simulink model "FOC08022311"  (R2025a)
settings: Solver=FixedStepAuto  StartTime=0.0  StopTime=1  RelTol=1e-3
values from neighbouring files (symbols this model uses):
  B = 0    [FOC08022311parameters.m]
  f_n = 50    [FOC08022311parameters.m]
  flux_n = L_m * Ids_n    [FOC08022311parameters.m]
  Ids_n = V_max / sqrt(R_s^2 + (w_n * L_s)^2)    [FOC08022311parameters.m]
  J = 0.1284    [FOC08022311parameters.m]
  ka_i = 1 / kp_i    (= 0.0140032473775)    [FOC08022311parameters.m]
  ki_i = R * wc_i    (= 19541.6337915)    [FOC08022311parameters.m]
  kp_i = L * wc_i    (= 71.4120070181)    [FOC08022311parameters.m]
  L_lr = 0.2898-0.2838    (= 0.006)    [FOC08022311parameters.m]
  L_ls = 0.294-0.2838    (= 0.0102)    [FOC08022311parameters.m]
  L_m = 1*0.2838    (= 0.2838)    [FOC08022311parameters.m]
  L_r = L_m + L_lr    (= 0.2898)    [FOC08022311parameters.m]
  L_s = L_m + L_ls    (= 0.294)    [FOC08022311parameters.m]
  n_p = 2    [FOC08022311parameters.m]
  P_n = 3000    [FOC08022311parameters.m]
  R_r = 2.658    [FOC08022311parameters.m]
  R_s = 1.85    [FOC08022311parameters.m]
  rpm_n = 1400    [FOC08022311parameters.m]
  sigma = 1 - L_m^2 / (L_s * L_r)    (= 0.0546795115562)    [FOC08022311parameters.m]
  T_r = L_r / R_r    (= 0.109029345372)    [FOC08022311parameters.m]
  T_sw = 1 / f_sw    (= 0.0001)    [FOC08022311parameters.m]
  V_dc = 500    [FOC08022311parameters.m]
  V_max = V_n * sqrt(2) / sqrt(3)    [FOC08022311parameters.m]
  V_n = 380    [FOC08022311parameters.m]
libraries: simulink x3, slpidlib x2, spsAsynchronousMachineSIUnitsLib x1, spsDCVoltageSourceLib x1, spsAlphaBetaZerotoabcLib x1, spsTriangleGeneratorLib x1, spsUniversalBridgeLib x1, spsabctodq0Lib x1, spsdq0toAlphaBetaZeroLib x1, spspowerguiLib x1
settings Model: Creator=11048  LastModifiedBy=ASUS
settings RTWCC: GPUComputeCapability=3.5

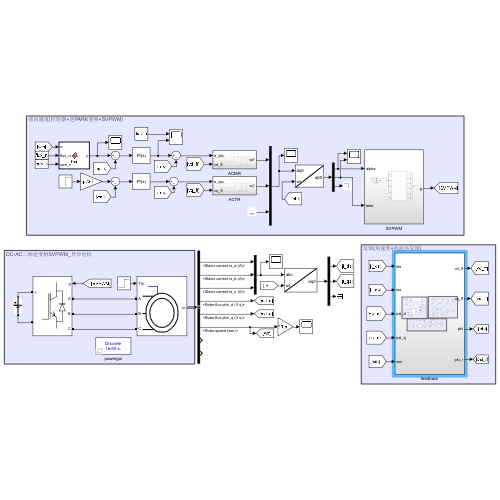
[thumbnail: Simulink's stored preview of the top-level diagram]
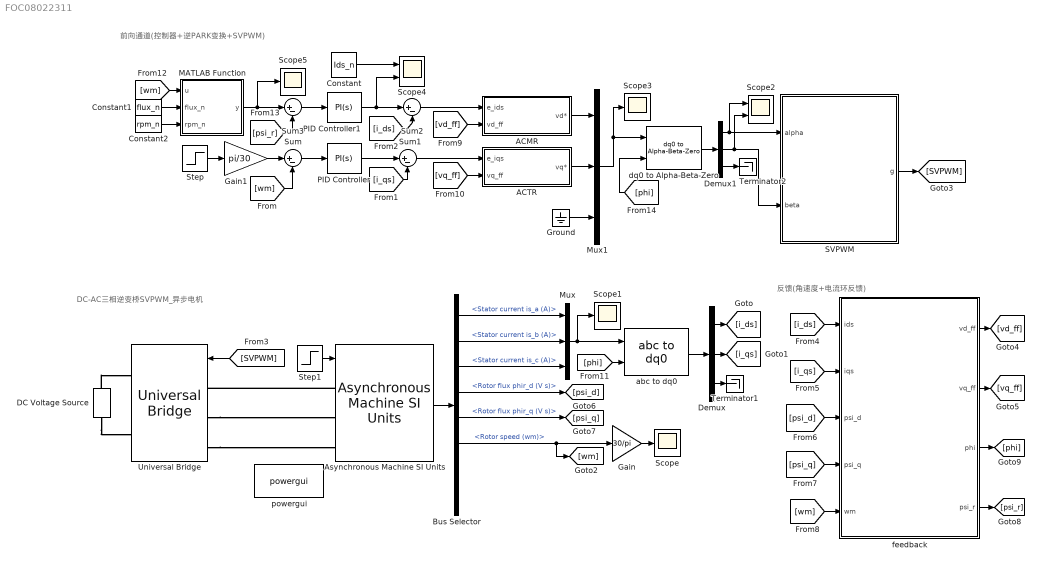
== system FOC08022311 ==
  note: 反馈(角速度+电流环反馈)
  note: 前向通道(控制器+逆PARK变换+SVPWM)
  note: DC-AC三相逆变桥SVPWM_异步电机
  ACMR : Subsystem
  ACTR : Subsystem
  Asynchronous Machine SI Units : spsAsynchronousMachineSIUnitsLib/Asynchronous Machine SI Units  RotorType=Squirrel-cage  PresetModel=No  MechanicalLoad=Torque Tm  ShowDetailedParameters=on  ReferenceFrame=Stationary  Units=SI  MeasurementBus=off  NominalParameters=[P_n V_n f_n]  VoltageRatio=1  Stator=[R_s L_ls]  Rotor=[R_r L_lr]  Cage1=[0.4155 0.002066]  Cage2=[0.4168 0.0003495]  Lm=L_m  Mechanical=[J B n_p]  PolePairs=2  InitialConditions=[1 0 0 0 0 0 0 0]  SimulateSaturation=off  Saturation=[14.03593122, 27.81365428, 53.79336849, 72.68890987, 97.98006896, 148.6815601, 215.7428561, 302.9841135, 428.7778367 ; 230, 322, 414, 460, 506, 552, 598, 644, 690]  LoadFlowParameters=1492000  TsPowergui=0  TsBlock=-1  IterativeModel=Trapezoidal non iterative  IterativeDiscreteModel=Trapezoidal non iterative  Pmec=1.492e+006
  Bus Selector : BusSelector  OutputSignals=Stator measurements.Stator current is_a (A),Stator measurements.Stator current is_b (A),Stator measurements.Stator current is_c (A),Rotor measurements.Rotor flux phir_d (V s),Rotor measurements.Rotor flux phir_q (V s),Mechanical.Rotor speed (wm),Mechanical.Electromagnetic torque Te (N*m),Mechanical.Rotor angle thetam (rad)
  Constant : Constant  Value=Ids_n
  Constant1 : Constant  Value=flux_n
  Constant2 : Constant  Value=rpm_n
  DC Voltage Source : spsDCVoltageSourceLib/DC Voltage Source  Amplitude=V_dc  Measurements=None
  Demux : Demux  Outputs=3
  Demux1 : Demux  Outputs=3
  Gain : Gain  Gain=30/pi
  Gain1 : Gain  Gain=pi/30
  Ground : Ground
  MATLAB Function : MATLAB Function  TreatAsAtomicUnit=on
  Mux : Mux  Inputs=3
  Mux1 : Mux  Inputs=3
  PID Controller : slpidlib/PID Controller  Controller=PI  Form=Parallel  TimeDomain=Continuous-time  UseExternalTs=off  SampleTime=-1  IntegratorMethod=Forward Euler  FilterMethod=Forward Euler  ControllerParametersSource=internal  P=20  I=1.5  UseKiTs=off  D=0  UseExternalDerivativeSource=off  N=100  UseFilter=on  TunerSelectOption=Transfer Function Based (PID Tuner App)  InitialConditionSource=internal  InitialConditionForIntegrator=0  InitialConditionForFilter=0  DifferentiatorICPrevScaledInput=0  ExternalReset=none  TrackingMode=off  Kt=1  LimitOutput=off  SatLimitsSource=internal  UpperSaturationLimit=inf  LowerSaturationLimit=-inf  LinearizeAsGain=on  AntiWindupMode=none  Kb=1  LimitIntegrator=off  UpperIntegratorSaturationLimit=inf  LowerIntegratorSaturationLimit=-inf  POutMin=[]  POutMax=[]  IOutMin=[]  IOutMax=[]  DOutMin=[]  DOutMax=[]  NOutMin=[]  NOutMax=[]  SumOutMin=[]  SumOutMax=[]  SaturationOutMin=[]  SaturationOutMax=[]  PParamMin=[]  PParamMax=[]  IParamMin=[]  IParamMax=[]  DParamMin=[]  DParamMax=[]  NParamMin=[]  NParamMax=[]  KbParamMin=[]  KbParamMax=[]  KtParamMin=[]  KtParamMax=[]  KbOutMin=[]  KbOutMax=[]  KtOutMin=[]  KtOutMax=[]  IntegratorOutMin=[]  IntegratorOutMax=[]  FilterOutMin=[]  FilterOutMax=[]  SumI1OutMin=[]  SumI1OutMax=[]  SumI2OutMin=[]  SumI2OutMax=[]  SumI3OutMin=[]  SumI3OutMax=[]  SumI4OutMin=[]  SumI4OutMax=[]  SumDOutMin=[]  SumDOutMax=[]  DifferentiatorOutMin=[]  DifferentiatorOutMax=[]  FilterDiffOutCoefMin=[]  FilterDiffOutCoefMax=[]  ReciprocalOutMin=[]  ReciprocalOutMax=[]  SumDenOutMin=[]  SumDenOutMax=[]  SumNumOutMin=[]  SumNumOutMax=[]  DivideOutMin=[]  DivideOutMax=[]  UdiffTsProdOutMin=[]  UdiffTsProdOutMax=[]  NTsProdOutMin=[]  NTsProdOutMax=[]  UintegralTsProdOutMin=[]  UintegralTsProdOutMax=[]  UngainTsProdOutMin=[]  UngainTsProdOutMax=[]  ClampingZeroOutDataTypeStr=Inherit: Inherit via back propagation  ClampingZeroOutMin=[]  ClampingZeroOutMax=[]  FilterDenConstantOutDataTypeStr=Inherit: Inherit via back propagation  FilterDenConstantOutMin=[]  FilterDenConstantOutMax=[]  PCopyOutDataTypeStr=Inherit: Inherit via back propagation  PCopyOutMin=[]  PCopyOutMax=[]  NCopyOutDataTypeStr=Inherit: Inherit via back propagation  NCopyOutMin=[]  NCopyOutMax=[]  IntegratorContinuousStateAttributes=''  IntegratorStateMustResolveToSignalObject=off  IntegratorRTWStateStorageClass=Auto  FilterContinuousStateAttributes=''  FilterStateMustResolveToSignalObject=off  FilterRTWStateStorageClass=Auto  ParallelPVariant=InternalParameters  IdealPVariant=Disabled  IVariant=InternalParameters  DVariant=Disabled  IntegratorVariant=Continuous  SatVariant=Disabled  AWVariant=Passthrough  PCopyVariant=Disabled  TRVariant=Disabled  FdbkBlocksVariant=Forward  IdealPFdbkVariant=Disabled  SatFdbkVariant=Disabled  DerivativeFilterVariant=Disabled  NVariant=Disabled  NCopyVariant=Disabled_SignalSpec  FilterICVariant=Disabled  IntegratorICVariant=InternalICs  ExternalResetVariant=Disabled  TRSumVariant=Passthrough  SumFdbkVariant=Disabled  SumVariant=Sum_PI  TsampFilterVariant=InternalTs  TsampNgainVariant=Passthrough  TsampIntegralVariant=Disabled_SignalSpec  ExternalSaturationOutDataTypeStr=Inherit: Same as second input  DerivativeSourceVariant=Disabled  PreIntVariant=InternalPreInt
  PID Controller1 : slpidlib/PID Controller  Controller=PI  Form=Parallel  TimeDomain=Continuous-time  UseExternalTs=off  SampleTime=-1  IntegratorMethod=Forward Euler  FilterMethod=Forward Euler  ControllerParametersSource=internal  P=1/L_m  I=5  UseKiTs=off  D=0  UseExternalDerivativeSource=off  N=100  UseFilter=on  TunerSelectOption=Transfer Function Based (PID Tuner App)  InitialConditionSource=internal  InitialConditionForIntegrator=0  InitialConditionForFilter=0  DifferentiatorICPrevScaledInput=0  ExternalReset=none  TrackingMode=off  Kt=1  LimitOutput=off  SatLimitsSource=internal  UpperSaturationLimit=inf  LowerSaturationLimit=-inf  LinearizeAsGain=on  AntiWindupMode=none  Kb=1  LimitIntegrator=off  UpperIntegratorSaturationLimit=inf  LowerIntegratorSaturationLimit=-inf  POutMin=[]  POutMax=[]  IOutMin=[]  IOutMax=[]  DOutMin=[]  DOutMax=[]  NOutMin=[]  NOutMax=[]  SumOutMin=[]  SumOutMax=[]  SaturationOutMin=[]  SaturationOutMax=[]  PParamMin=[]  PParamMax=[]  IParamMin=[]  IParamMax=[]  DParamMin=[]  DParamMax=[]  NParamMin=[]  NParamMax=[]  KbParamMin=[]  KbParamMax=[]  KtParamMin=[]  KtParamMax=[]  KbOutMin=[]  KbOutMax=[]  KtOutMin=[]  KtOutMax=[]  IntegratorOutMin=[]  IntegratorOutMax=[]  FilterOutMin=[]  FilterOutMax=[]  SumI1OutMin=[]  SumI1OutMax=[]  SumI2OutMin=[]  SumI2OutMax=[]  SumI3OutMin=[]  SumI3OutMax=[]  SumI4OutMin=[]  SumI4OutMax=[]  SumDOutMin=[]  SumDOutMax=[]  DifferentiatorOutMin=[]  DifferentiatorOutMax=[]  FilterDiffOutCoefMin=[]  FilterDiffOutCoefMax=[]  ReciprocalOutMin=[]  ReciprocalOutMax=[]  SumDenOutMin=[]  SumDenOutMax=[]  SumNumOutMin=[]  SumNumOutMax=[]  DivideOutMin=[]  DivideOutMax=[]  UdiffTsProdOutMin=[]  UdiffTsProdOutMax=[]  NTsProdOutMin=[]  NTsProdOutMax=[]  UintegralTsProdOutMin=[]  UintegralTsProdOutMax=[]  UngainTsProdOutMin=[]  UngainTsProdOutMax=[]  ClampingZeroOutDataTypeStr=Inherit: Inherit via back propagation  ClampingZeroOutMin=[]  ClampingZeroOutMax=[]  FilterDenConstantOutDataTypeStr=Inherit: Inherit via back propagation  FilterDenConstantOutMin=[]  FilterDenConstantOutMax=[]  PCopyOutDataTypeStr=Inherit: Inherit via back propagation  PCopyOutMin=[]  PCopyOutMax=[]  NCopyOutDataTypeStr=Inherit: Inherit via back propagation  NCopyOutMin=[]  NCopyOutMax=[]  IntegratorContinuousStateAttributes=''  IntegratorStateMustResolveToSignalObject=off  IntegratorRTWStateStorageClass=Auto  FilterContinuousStateAttributes=''  FilterStateMustResolveToSignalObject=off  FilterRTWStateStorageClass=Auto  ParallelPVariant=InternalParameters  IdealPVariant=Disabled  IVariant=InternalParameters  DVariant=Disabled  IntegratorVariant=Continuous  SatVariant=Disabled  AWVariant=Passthrough  PCopyVariant=Disabled  TRVariant=Disabled  FdbkBlocksVariant=Forward  IdealPFdbkVariant=Disabled  SatFdbkVariant=Disabled  DerivativeFilterVariant=Disabled  NVariant=Disabled  NCopyVariant=Disabled_SignalSpec  FilterICVariant=Disabled  IntegratorICVariant=InternalICs  ExternalResetVariant=Disabled  TRSumVariant=Passthrough  SumFdbkVariant=Disabled  SumVariant=Sum_PI  TsampFilterVariant=InternalTs  TsampNgainVariant=Passthrough  TsampIntegralVariant=Disabled_SignalSpec  ExternalSaturationOutDataTypeStr=Inherit: Same as second input  DerivativeSourceVariant=Disabled  PreIntVariant=InternalPreInt
  SVPWM : Subsystem
  Scope{,1,3,5} (4 alike) : Scope
      Scope settings: ActiveDisplayYMinimum=-245.05423330740308  ActiveDisplayYMaximum=2182.1289862079198
      Scope1 settings: ActiveDisplayYMinimum=-1  ActiveDisplayYMaximum=1  DataLoggingVariableName=ScopeData2
      Scope3 settings: ActiveDisplayYMinimum=-553.80143526649249  ActiveDisplayYMaximum=499.74368491943784
      Scope5 settings: ActiveDisplayYMinimum=0.877559064610581  ActiveDisplayYMaximum=0.96156070598738208  DataLoggingVariableName=ScopeData9
  Scope2 : Scope  NumInputPorts=2
      settings: ActiveDisplayYMinimum=-1  ActiveDisplayYMaximum=1  DataLoggingVariableName=ScopeData5
  Scope4 : Scope  NumInputPorts=2
      settings: ActiveDisplayYMinimum=-2.7427305612345254  ActiveDisplayYMaximum=4.03663172867287  DataLoggingVariableName=ScopeData8
  Step : Step  Time=0.6  Before=1000  After=1500  SampleTime=0
  Step1 : Step  Time=0.3  Before=10  After=20  SampleTime=0
  Sum{,1..3} (4 alike) : Sum  Inputs=|+-
  Terminator1 : Terminator
  Terminator2 : Terminator
  Universal Bridge : spsUniversalBridgeLib/Universal Bridge  Arms=3  SnubberResistance=1e5  SnubberCapacitance=inf  Device=IGBT / Diodes  Ron=1e-3  Lon=0  ForwardVoltages="[  0  0  ]"  ForwardVoltage=0  GTOparameters=[ 10e-6 , 20e-6 ]  IGBTparameters=[ 1e-6 , 2e-6 ]  Measurements=None  Measurements_2=None  converterType=Rectifier
  abc to dq0 : spsabctodq0Lib/abc to dq0  Alignment=90 degrees behind phase A axis
  dq0 to Alpha-Beta-Zero : spsdq0toAlphaBetaZeroLib/dq0 to Alpha-Beta-Zero  Alignment=90 degrees behind phase A axis
  feedback : Subsystem
  powergui : spspowerguiLib/powergui  Priority=1  SimulationMode=Discrete  SampleTime=T_sw/10  frequency=60  Iterations=50  frequencyindice=50  Pbase=100e6  ErrMax=1e-4  UnitsV=kV  UnitsW=MW  buscounter=0  FunctionMessages=off  echomessages=off  EnableUseOfTLC=off  CurrentSourceSwitches=off  DisableSnubberDevices=off  DisableRonSwitches=off  DisableVfSwitches=off  DisplayEquations=off  AutomaticDiscreteSolvers=off  SolverType=Tustin/Backward Euler (TBE)  Interpol=off  ExternalGateDelay=off  methode=off  Ts=100  x0status=blocks  SPID=on  SwTol=0  HookPort=off  NonlinearTolerance=1e-4  nMaxIteration=100  ContinueOnMaxIteration=off  RestoreLinks=warning  ResistiveCurrentMeasurement=off  Frange=[0:2:500]  Ylog=off  Xlog=on  ShowGrid=off  save=off  variable=ZData  structure=0  ZoomFFT=off  StartTime=0.0  cycles=1  DisplayStyle=1  fundamental=60  FreqAxis=off  MaxFrequency=1000  frequencyindicesteady=1  RmsSteady=1  display=off
  wires:
  Asynchronous Machine SI Units/1 -> Bus Selector/1
  Bus Selector/4 -> [psi_d]  "<Rotor flux phir_d (V s)>"
  Bus Selector/1 -> Mux/1  "<Stator current is_a (A)>"
  Bus Selector/2 -> Mux/2  "<Stator current is_b (A)>"
  Bus Selector/3 -> Mux/3  "<Stator current is_c (A)>"
  Bus Selector/6 -> Gain/1, [wm]  "<Rotor speed (wm)>"
  Gain/1 -> Scope/1
  Step/1 -> Gain1/1
  Gain1/1 -> Sum/1
  [wm] -> Sum/2
  Sum/1 -> PID Controller/1
  PID Controller/1 -> Sum1/1
  [i_qs] -> Sum1/2
  Sum1/1 -> ACTR/1(e_iqs)
  [i_ds] -> Sum2/2
  Sum2/1 -> ACMR/1(e_ids)
  Mux1/1 -> dq0 to Alpha-Beta-Zero/1, Scope3/1
  dq0 to Alpha-Beta-Zero/1 -> Demux1/1
  Demux1/3 -> Terminator2/1
  [SVPWM] -> Universal Bridge/1
  feedback/2(vq_ff) -> [vq_ff]
  [i_qs] -> feedback/2(iqs)
  [psi_d] -> feedback/3(psi_d)
  [psi_q] -> feedback/4(psi_q)
  [wm] -> feedback/5(wm)
  [vq_ff] -> ACTR/2(vq_ff)
  [vd_ff] -> ACMR/2(vd_ff)
  Step1/1 -> Asynchronous Machine SI Units/1
  SVPWM/1(g) -> [SVPWM]
  Demux/3 -> Terminator1/1
  Demux/1 -> [i_ds]
  Demux/2 -> [i_qs]
  abc to dq0/1 -> Demux/1
  [phi] -> abc to dq0/2
  Mux/1 -> abc to dq0/1, Scope1/1
  Bus Selector/5 -> [psi_q]  "<Rotor flux phir_q (V s)>"
  [i_ds] -> feedback/1(ids)
  [phi] -> dq0 to Alpha-Beta-Zero/2
  Demux1/1 -> SVPWM/1(alpha), Scope2/1
  Demux1/2 -> SVPWM/2(beta), Scope2/2
  feedback/3(phi) -> [phi]
  Ground/1 -> Mux1/3
  ACMR/1(vd*) -> Mux1/1
  ACTR/1(vq*) -> Mux1/2
  feedback/1(vd_ff) -> [vd_ff]
  PID Controller1/1 -> Scope4/2, Sum2/1
  [wm] -> MATLAB Function/1(u)
  feedback/4(psi_r) -> [psi_r]
  [psi_r] -> Sum3/2
  MATLAB Function/1(y) -> Scope5/1, Sum3/1
  Sum3/1 -> PID Controller1/1
  Constant1/1 -> MATLAB Function/2(flux_n)
  Constant2/1 -> MATLAB Function/3(rpm_n)
  Constant/1 -> Scope4/1
  connections:
  DC Voltage Source/RConn1 -- Universal Bridge/RConn1
  DC Voltage Source/LConn1 -- Universal Bridge/RConn2
  Asynchronous Machine SI Units/LConn1 -- Universal Bridge/LConn1
  Universal Bridge/LConn2 -- Asynchronous Machine SI Units/LConn2
  Universal Bridge/LConn3 -- Asynchronous Machine SI Units/LConn3

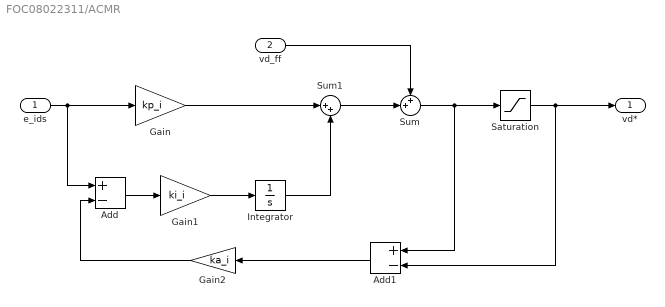
== system FOC08022311/ACMR ==
  e_ids : Inport
  vd_ff : Inport  Port=2
  Add : Sum  Inputs=+-
  Add1 : Sum  Inputs=+-
  Gain : Gain  Gain=kp_i
  Gain1 : Gain  Gain=ki_i
  Gain2 : Gain  Gain=ka_i
  Integrator : Integrator
  Saturation : Saturate  UpperLimit=V_max * 2  LowerLimit=-V_max * 2
  Sum : Sum  Inputs=++|
  Sum1 : Sum  Inputs=|++
  vd* : Outport
  wires:
  Gain2/1 -> Add/2
  Add1/1 -> Gain2/1
  Saturation/1 -> vd*/1, Add1/2
  Sum/1 -> Saturation/1, Add1/1
  Add/1 -> Gain1/1
  e_ids/1 -> Add/1, Gain/1
  vd_ff/1 -> Sum/1
  Integrator/1 -> Sum1/2
  Gain/1 -> Sum1/1
  Sum1/1 -> Sum/2
  Gain1/1 -> Integrator/1

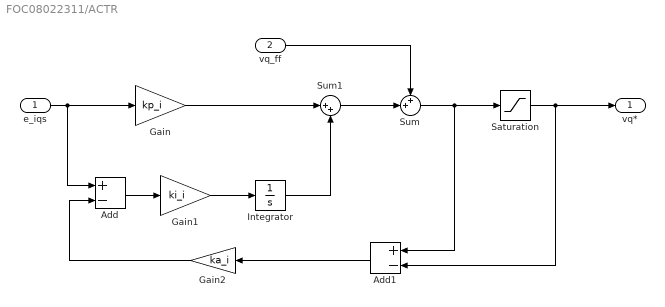
== system FOC08022311/ACTR ==
  e_iqs : Inport
  vq_ff : Inport  Port=2
  Add : Sum  Inputs=+-
  Add1 : Sum  Inputs=+-
  Gain : Gain  Gain=kp_i
  Gain1 : Gain  Gain=ki_i
  Gain2 : Gain  Gain=ka_i
  Integrator : Integrator
  Saturation : Saturate  UpperLimit=V_max*2  LowerLimit=-V_max * 2
  Sum : Sum  Inputs=++|
  Sum1 : Sum  Inputs=|++
  vq* : Outport
  wires:
  Gain1/1 -> Integrator/1
  Sum1/1 -> Sum/2
  Gain/1 -> Sum1/1
  Integrator/1 -> Sum1/2
  vq_ff/1 -> Sum/1
  e_iqs/1 -> Gain/1, Add/1
  Add/1 -> Gain1/1
  Sum/1 -> Add1/1, Saturation/1
  Saturation/1 -> Add1/2, vq*/1
  Add1/1 -> Gain2/1
  Gain2/1 -> Add/2

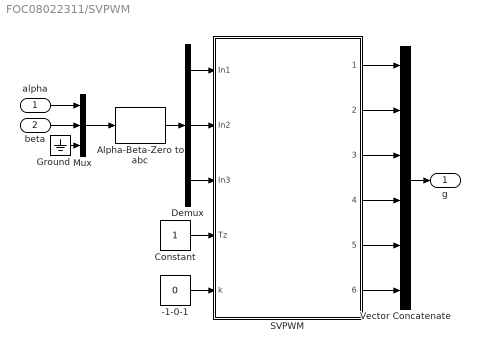
== system FOC08022311/SVPWM ==
  alpha : Inport
  beta : Inport  Port=2
  -1-0-1 : Constant  Value=0
  Alpha-Beta-Zero to abc : spsAlphaBetaZerotoabcLib/Alpha-Beta-Zero to abc
      settings: LibrarySourceBlock=|
      | sps_lib/Control/Alpha-Beta-Zero
      | to abc
  Constant : Constant
  Demux : Demux  Outputs=3
  Ground : Ground
  Mux : Mux  Inputs=3
  SVPWM : Subsystem
  Vector Concatenate : Concatenate  NumInputs=6
  g : Outport
  wires:
  alpha/1 -> Mux/1
  beta/1 -> Mux/2
  SVPWM/5(5) -> Vector Concatenate/5
  SVPWM/4(4) -> Vector Concatenate/4
  Demux/2 -> SVPWM/2(In2)
  -1-0-1/1 -> SVPWM/5(k)
  SVPWM/6(6) -> Vector Concatenate/6
  Constant/1 -> SVPWM/4(Tz)
  SVPWM/2(2) -> Vector Concatenate/2
  Demux/3 -> SVPWM/3(In3)
  SVPWM/1(1) -> Vector Concatenate/1
  Demux/1 -> SVPWM/1(In1)
  SVPWM/3(3) -> Vector Concatenate/3
  Vector Concatenate/1 -> g/1
  Mux/1 -> Alpha-Beta-Zero to abc/1
  Alpha-Beta-Zero to abc/1 -> Demux/1
  Ground/1 -> Mux/3

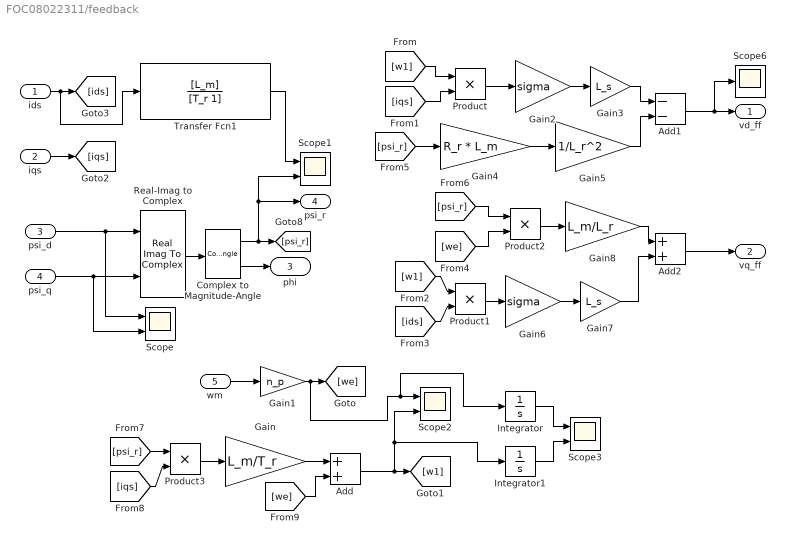
== system FOC08022311/feedback ==
  ids : Inport
  iqs : Inport  Port=2
  psi_d : Inport  Port=3
  psi_q : Inport  Port=4
  wm : Inport  Port=5
  Add : Sum
  Add1 : Sum  Inputs=--
  Add2 : Sum
  Complex to Magnitude-Angle : ComplexToMagnitudeAngle
  Gain : Gain  Gain=L_m/T_r
  Gain1 : Gain  Gain=n_p
  Gain2 : Gain  Gain=sigma
  Gain3 : Gain  Gain=L_s
  Gain4 : Gain  Gain=R_r * L_m
  Gain5 : Gain  Gain=1/L_r^2
  Gain6 : Gain  Gain=sigma
  Gain7 : Gain  Gain=L_s
  Gain8 : Gain  Gain=L_m/L_r
  Integrator : Integrator
  Integrator1 : Integrator
  Product{,1..3} (4 alike) : Product
  Real-Imag to Complex : RealImagToComplex
  Scope{,1..3} (4 alike) : Scope  NumInputPorts=2
      Scope settings: ActiveDisplayYMinimum=-1.6110842776276593  ActiveDisplayYMaximum=1.5992338688221852  DataLoggingVariableName=ScopeData7
      Scope1 settings: ActiveDisplayYMinimum=-0.19199842830712538  ActiveDisplayYMaximum=1.7279858547641289  DataLoggingVariableName=ScopeData3
      Scope2 settings: ActiveDisplayYMinimum=-28.950143898994849  ActiveDisplayYMaximum=260.34761589561333  DataLoggingVariableName=ScopeData4
      Scope3 settings: ActiveDisplayYMinimum=-1  ActiveDisplayYMaximum=1  DataLoggingVariableName=ScopeData6
  Scope6 : Scope
      settings: ActiveDisplayYMinimum=-1  ActiveDisplayYMaximum=1  DataLoggingVariableName=usm0601  DataLoggingSaveFormat=Array
  Transfer Fcn1 : TransferFcn  Numerator=[L_m]  Denominator=[T_r 1]
  vd_ff : Outport
  vq_ff : Outport  Port=2
  phi : Outport  Port=3
  psi_r : Outport  Port=4
  wires:
  ids/1 -> Transfer Fcn1/1, [ids]
  iqs/1 -> [iqs]
  Gain/1 -> Add/1
  wm/1 -> Gain1/1
  Gain1/1 -> Integrator/1, Scope2/1, [we]
  Add/1 -> Integrator1/1, Scope2/2, [w1]
  [w1] -> Product/1
  [iqs] -> Product/2
  Product/1 -> Gain2/1
  Gain2/1 -> Gain3/1
  Gain4/1 -> Gain5/1
  Gain3/1 -> Add1/1
  Gain5/1 -> Add1/2
  Add1/1 -> vd_ff/1, Scope6/1
  Gain6/1 -> Gain7/1
  [w1] -> Product1/1
  Product1/1 -> Gain6/1
  [ids] -> Product1/2
  [we] -> Product2/2
  Product2/1 -> Gain8/1
  Gain8/1 -> Add2/1
  Gain7/1 -> Add2/2
  Add2/1 -> vq_ff/1
  psi_d/1 -> Real-Imag to Complex/1, Scope/1
  Real-Imag to Complex/1 -> Complex to Magnitude-Angle/1
  Complex to Magnitude-Angle/2 -> phi/1
  Complex to Magnitude-Angle/1 -> psi_r/1, Scope1/2, [psi_r]
  psi_q/1 -> Scope/2, Real-Imag to Complex/2
  Product3/1 -> Gain/1
  [psi_r] -> Gain4/1
  [psi_r] -> Product2/1
  [psi_r] -> Product3/1
  [iqs] -> Product3/2
  [we] -> Add/2
  Transfer Fcn1/1 -> Scope1/1
  Integrator/1 -> Scope3/1
  Integrator1/1 -> Scope3/2

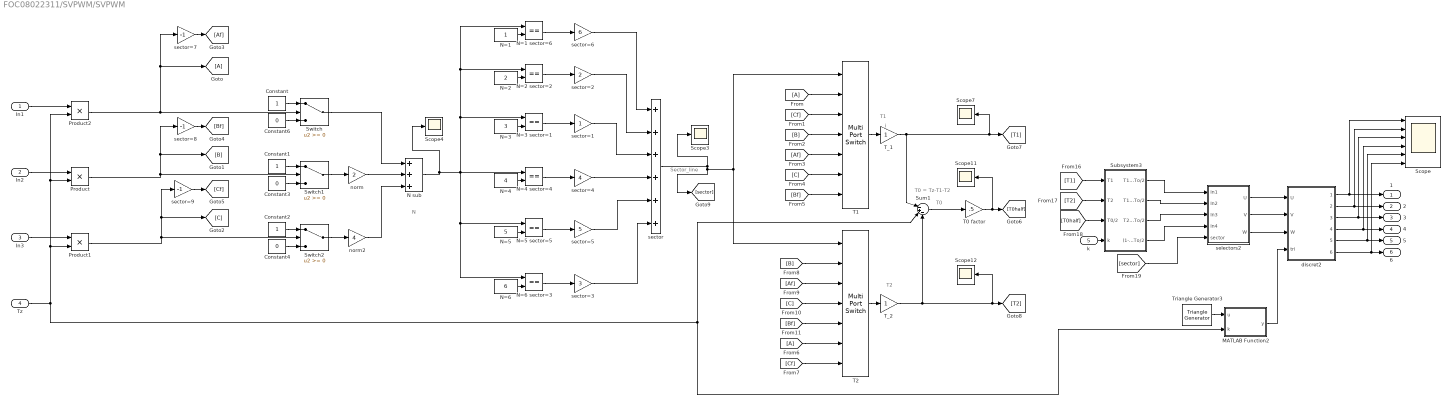
== system FOC08022311/SVPWM/SVPWM ==
  note: T1
  note: T2
  note: i
  note: N
  note: T0 = Tz-T1-T2
  note: Sector_line
  note: T0
  In1 : Inport
  In2 : Inport  Port=2
  In3 : Inport  Port=3
  Tz : Inport  Port=4
  k : Inport  Port=5
  Constant : Constant
  Constant1 : Constant
  Constant2 : Constant
  Constant3 : Constant  Value=0
  Constant4 : Constant  Value=0
  Constant6 : Constant  Value=0
  From : From
  From6 : From
  Goto : Goto
  MATLAB Function2 : MATLAB Function  TreatAsAtomicUnit=on
  N sub : Sum  Inputs=+++
  N=1 : Constant
  N=1 sector=6 : RelationalOperator  Operator===  OutDataTypeStr=boolean  InputSameDT=off
  N=2 : Constant  Value=2
  N=2 sector=2 : RelationalOperator  Operator===  OutDataTypeStr=boolean  InputSameDT=off
  N=3 : Constant  Value=3
  N=3 sector=1 : RelationalOperator  Operator===  OutDataTypeStr=boolean  InputSameDT=off
  N=4 : Constant  Value=4
  N=4 sector=4 : RelationalOperator  Operator===  OutDataTypeStr=boolean  InputSameDT=off
  N=5 : Constant  Value=5
  N=5 sector=5 : RelationalOperator  Operator===  OutDataTypeStr=boolean  InputSameDT=off
  N=6 : Constant  Value=6
  N=6 sector=3 : RelationalOperator  Operator===  OutDataTypeStr=boolean  InputSameDT=off
  Product : Product
  Product1 : Product
  Product2 : Product
  Scope : Scope  NumInputPorts=6
      settings: ActiveDisplayYMinimum=-0.11983471074380159  ActiveDisplayYMaximum=1.0733471074380165
  Scope{3..4,7,11..12} (5 alike) : Scope
      Scope11 settings: ActiveDisplayYMinimum=-492.93722989300011  ActiveDisplayYMaximum=53.609603972290969  DataLoggingVariableName=current2
      Scope12 settings: ActiveDisplayYMinimum=-47.570247237341619  ActiveDisplayYMaximum=581.67686973428681  DataLoggingVariableName=current3
      Scope3 settings: ActiveDisplayYMinimum=0.81076195805055384  ActiveDisplayYMaximum=6.2254857247595474  DataLoggingVariableName=ScopeData3
      Scope4 settings: ActiveDisplayYMinimum=0.33967719556370923  ActiveDisplayYMaximum=7.0888774478654026  DataLoggingVariableName=ScopeData4
      Scope7 settings: ActiveDisplayYMinimum=-744.74431123189447  ActiveDisplayYMaximum=933.20587173538911  DataLoggingVariableName=current1
  Subsystem3 : Subsystem
  Sum1 : Sum  Inputs=|-+-
  Switch : Switch  SaturateOnIntegerOverflow=off  InputSameDT=off
  Switch1 : Switch  SaturateOnIntegerOverflow=off  InputSameDT=off
  Switch2 : Switch  SaturateOnIntegerOverflow=off  InputSameDT=off
  T0 factor : Gain  Gain=.5
  T1 : MultiPortSwitch  DataPortOrder=Specify indices  Inputs=4  DataPortIndices={1,2,3,4,5,6}  DiagnosticForDefault=None  SaturateOnIntegerOverflow=off  InputSameDT=off
  T2 : MultiPortSwitch  DataPortOrder=Specify indices  Inputs=4  DataPortIndices={1,2,3,4,5,6}  DiagnosticForDefault=None  SaturateOnIntegerOverflow=off  InputSameDT=off
  T_1 : Gain
  T_2 : Gain
  Triangle Generator3 : spsTriangleGeneratorLib/Triangle Generator  Freq=50e3  Phase=180  Ts=0
  discret2 : Subsystem
  norm : Gain  Gain=2
  norm2 : Gain  Gain=4
  sector : Sum  Inputs=++++++
  sector=1 : Gain
  sector=2 : Gain  Gain=2
  sector=3 : Gain  Gain=3
  sector=4 : Gain  Gain=4
  sector=5 : Gain  Gain=5
  sector=6 : Gain  Gain=6
  sector=7 : Gain  Gain=-1
  sector=8 : Gain  Gain=-1
  sector=9 : Gain  Gain=-1
  selectors2 : Subsystem
  1 : Outport
  2 : Outport  Port=2
  3 : Outport  Port=3
  4 : Outport  Port=4
  5 : Outport  Port=5
  6 : Outport  Port=6
  wires:
  Subsystem3/1(T1+T2+(1-k)To/2) -> selectors2/1(In1)
  selectors2/2(V) -> discret2/2(V)
  [T0half] -> Subsystem3/3(T0/2)
  [T1] -> Subsystem3/1(T1)
  Subsystem3/2(T1+(1-k)To/2) -> selectors2/2(In2)
  [sector] -> selectors2/5("sector ")
  MATLAB Function2/1(y) -> discret2/4(tri)
  [T2] -> Subsystem3/2(T2)
  selectors2/1(U) -> discret2/1(U)
  Triangle Generator3/1 -> MATLAB Function2/1(u)
  selectors2/3(W) -> discret2/3(W)
  Subsystem3/3(T2+(1-k)To/2) -> selectors2/3(In3)
  k/1 -> Subsystem3/4(k)
  discret2/1(1) -> Scope/1, 1/1
  discret2/6(6) -> Scope/6, 6/1
  discret2/2(2) -> Scope/2, 2/1
  discret2/3(3) -> Scope/3, 3/1
  discret2/5(5) -> Scope/5, 5/1
  discret2/4(4) -> Scope/4, 4/1
  T_1/1 -> Scope7/1, [T1], Sum1/1
  sector=4/1 -> sector/4
  N sub/1 -> N=6 sector=3/1, N=5 sector=5/1, N=4 sector=4/1, N=3 sector=1/1, N=1 sector=6/1, N=2 sector=2/1, Scope4/1
  Subsystem3/4((1-k)To/2) -> selectors2/4(In4)
  [Af] -> T2/3
  T_2/1 -> Scope12/1, [T2], Sum1/3
  Tz/1 -> Product/2, Product2/2, Product1/2, Sum1/2, MATLAB Function2/2(k)
  T2/1 -> T_2/1
  norm2/1 -> N sub/3
  [C] -> T1/6
  [B] -> T2/2
  sector=9/1 -> [Cf]
  sector=7/1 -> [Af]
  sector/1 -> [sector], T2/1, T1/1, Scope3/1
  [Bf] -> T2/5
  norm/1 -> N sub/2
  sector=8/1 -> [Bf]
  [Cf] -> T1/3
  N=3 sector=1/1 -> sector=1/1
  [Cf] -> T2/7
  Constant6/1 -> Switch/3
  Sum1/1 -> T0 factor/1
  [Bf] -> T1/7
  From6/1 -> T2/6
  N=6 sector=3/1 -> sector=3/1
  sector=5/1 -> sector/5
  Switch2/1 -> norm2/1
  N=4/1 -> N=4 sector=4/2
  N=2/1 -> N=2 sector=2/2
  Constant/1 -> Switch/1
  sector=6/1 -> sector/1
  N=5/1 -> N=5 sector=5/2
  N=3/1 -> N=3 sector=1/2
  N=2 sector=2/1 -> sector=2/1
  [Af] -> T1/5
  [C] -> T2/4
  sector=2/1 -> sector/2
  sector=1/1 -> sector/3
  N=1 sector=6/1 -> sector=6/1
  sector=3/1 -> sector/6
  T1/1 -> T_1/1
  N=4 sector=4/1 -> sector=4/1
  Switch1/1 -> norm/1
  N=6/1 -> N=6 sector=3/2
  From/1 -> T1/2
  Switch/1 -> N sub/1
  N=5 sector=5/1 -> sector=5/1
  [B] -> T1/4
  T0 factor/1 -> Scope11/1, [T0half]
  Product/1 -> sector=8/1, [B], Switch1/2
  Product2/1 -> sector=7/1, Goto/1, Switch/2
  In1/1 -> Product2/1
  In3/1 -> Product1/1
  In2/1 -> Product/1
  Product1/1 -> sector=9/1, [C], Switch2/2
  Constant1/1 -> Switch1/1
  Constant2/1 -> Switch2/1
  Constant3/1 -> Switch1/3
  Constant4/1 -> Switch2/3
  N=1/1 -> N=1 sector=6/2

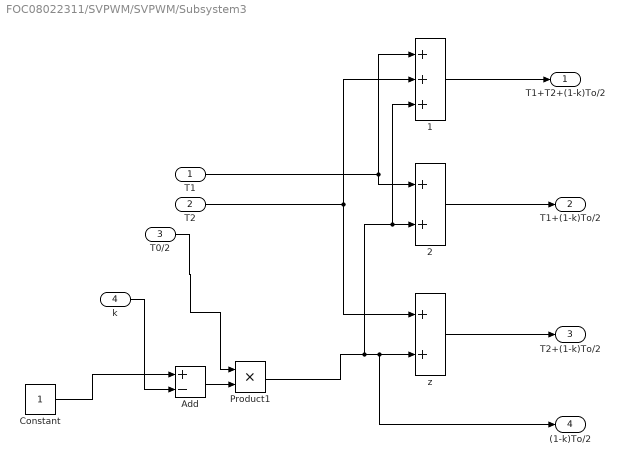
== system FOC08022311/SVPWM/SVPWM/Subsystem3 ==
  T1 : Inport
  T2 : Inport  Port=2
  T0/2 : Inport  Port=3
  k : Inport  Port=4
  1 : Sum  Inputs=+++
  2 : Sum
  Add : Sum  Inputs=+-
  Constant : Constant
  Product1 : Product
  z : Sum
  T1+T2+(1-k)To/2 : Outport
  T1+(1-k)To/2 : Outport  Port=2
  T2+(1-k)To/2 : Outport  Port=3
  (1-k)To/2 : Outport  Port=4
  wires:
  T1/1 -> 2/1, 1/1
  T0/2/1 -> Product1/1
  2/1 -> T1+(1-k)To/2/1
  1/1 -> T1+T2+(1-k)To/2/1
  T2/1 -> z/1, 1/2
  z/1 -> T2+(1-k)To/2/1
  Constant/1 -> Add/1
  k/1 -> Add/2
  Add/1 -> Product1/2
  Product1/1 -> 1/3, 2/2, (1-k)To/2/1, z/2

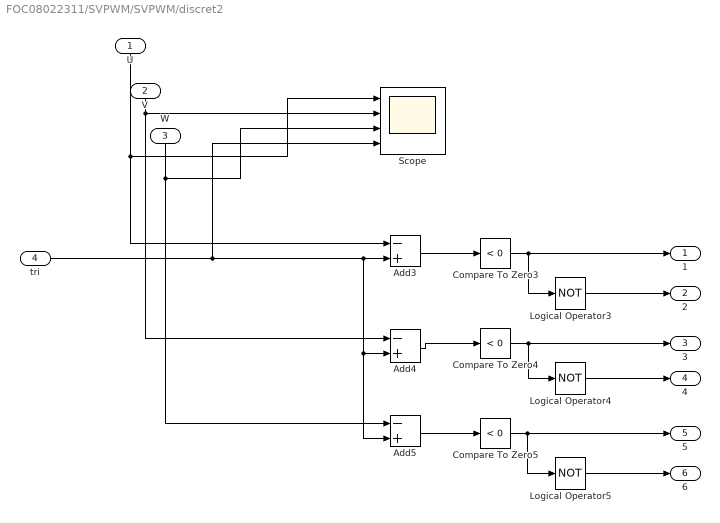
== system FOC08022311/SVPWM/SVPWM/discret2 ==
  U : Inport
  V : Inport  Port=2
  W : Inport  Port=3
  tri : Inport  Port=4
  Add3 : Sum  Inputs=-+
  Add4 : Sum  Inputs=-+
  Add5 : Sum  Inputs=-+
  Compare To Zero3 : simulink/Logic and Bit Operations/Compare To Zero  relop=<  OutDataTypeStr=boolean
  Compare To Zero4 : simulink/Logic and Bit Operations/Compare To Zero  relop=<  OutDataTypeStr=boolean
  Compare To Zero5 : simulink/Logic and Bit Operations/Compare To Zero  relop=<  OutDataTypeStr=boolean
  Logical Operator3 : Logic  Operator=NOT  AllPortsSameDT=off  OutDataTypeStr=boolean
  Logical Operator4 : Logic  Operator=NOT  AllPortsSameDT=off  OutDataTypeStr=boolean
  Logical Operator5 : Logic  Operator=NOT  AllPortsSameDT=off  OutDataTypeStr=boolean
  Scope : Scope  NumInputPorts=4
      settings: ActiveDisplayYMinimum=-546.26196625582566  ActiveDisplayYMaximum=533.53223123772113  DataLoggingVariableName=ScopeData2
  1 : Outport
  2 : Outport  Port=2
  3 : Outport  Port=3
  4 : Outport  Port=4
  5 : Outport  Port=5
  6 : Outport  Port=6
  wires:
  Compare To Zero4/1 -> Logical Operator4/1, 3/1
  Compare To Zero5/1 -> Logical Operator5/1, 5/1
  Logical Operator3/1 -> 2/1
  Compare To Zero3/1 -> Logical Operator3/1, 1/1
  Logical Operator4/1 -> 4/1
  Logical Operator5/1 -> 6/1
  V/1 -> Scope/2, Add4/1
  W/1 -> Scope/3, Add5/1
  U/1 -> Scope/1, Add3/1
  Add5/1 -> Compare To Zero5/1
  Add3/1 -> Compare To Zero3/1
  Add4/1 -> Compare To Zero4/1
  tri/1 -> Scope/4, Add3/2, Add5/2, Add4/2

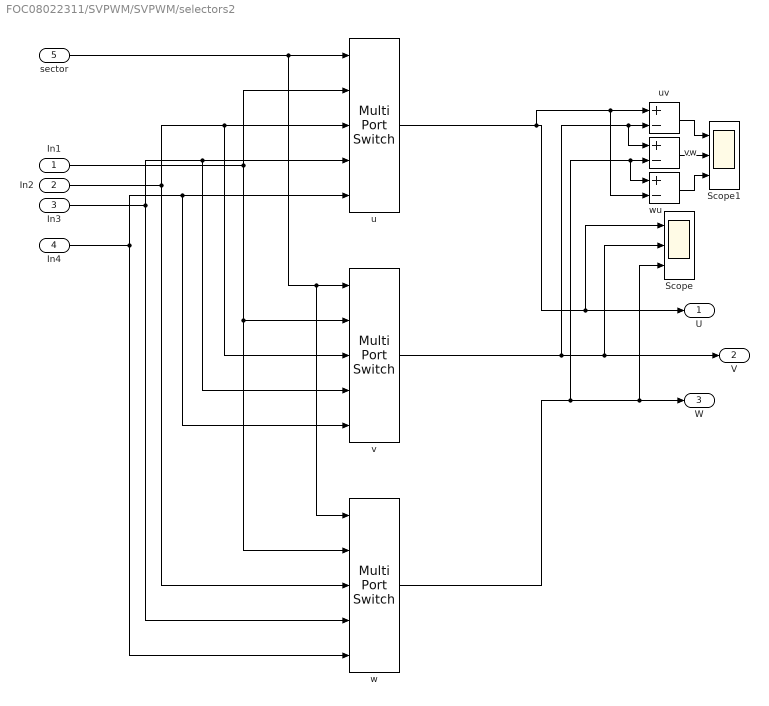
== system FOC08022311/SVPWM/SVPWM/selectors2 ==
  In1 : Inport
  In2 : Inport  Port=2
  In3 : Inport  Port=3
  In4 : Inport  Port=4
  "sector " : Inport  Port=5
  Scope : Scope  NumInputPorts=3
      settings: ActiveDisplayYMinimum=-0.125  ActiveDisplayYMaximum=1.125
  Scope1 : Scope  NumInputPorts=3
      settings: ActiveDisplayYMinimum=-1.25  ActiveDisplayYMaximum=1.25  DataLoggingVariableName=ScopeData6
  u : MultiPortSwitch  DataPortOrder=Specify indices  Inputs=4  DataPortIndices={[1,6],2,5,[3,4]}  DiagnosticForDefault=None  SaturateOnIntegerOverflow=off  InputSameDT=off
  uv : Sum  Inputs=+-
  v : MultiPortSwitch  DataPortOrder=Specify indices  Inputs=4  DataPortIndices={[2,3],4,1,[5,6]}  DiagnosticForDefault=None  SaturateOnIntegerOverflow=off  InputSameDT=off
  vw : Sum  Inputs=+-
  w : MultiPortSwitch  DataPortOrder=Specify indices  Inputs=4  DataPortIndices={[4,5],6,3,[1,2]}  DiagnosticForDefault=None  SaturateOnIntegerOverflow=off  InputSameDT=off
  wu : Sum  Inputs=+-
  U : Outport
  V : Outport  Port=2
  W : Outport  Port=3
  wires:
  u/1 -> wu/2, uv/1, Scope/1, U/1
  In1/1 -> v/2, w/2, u/2
  In2/1 -> w/3, u/3, v/3
  w/1 -> wu/1, vw/2, Scope/3, W/1
  In3/1 -> w/4, u/4, v/4
  v/1 -> vw/1, uv/2, Scope/2, V/1
  "sector "/1 -> w/1, v/1, u/1
  vw/1 -> Scope1/2
  uv/1 -> Scope1/1
  wu/1 -> Scope1/3
  In4/1 -> w/5, u/5, v/5

== matlab function FOC08022311/SVPWM/SVPWM/MATLAB Function2 ==
  data: u input; y output; k input
function y = fcn(u,k)
% y = k*(u+1)/2;
y=k*u;

== matlab function FOC08022311/MATLAB Function ==
  data: u input; y output; flux_n input; rpm_n input
function y = fcn(u,flux_n,rpm_n)
if u<(rpm_n*pi/30)
    y=flux_n;
else
    y=flux_n*(rpm_n*pi/30)/u;
end
